simulink model "task1_sim"  (R2024a)
settings: Solver=VariableStepAuto  StartTime=0.0  StopTime=10.0  RelTol=1e-3
values from neighbouring files (symbols this model uses):
  a = zad1.a    [initilize_task1.m]    (also in task1.m; task1_1.m; task1_2.m; task1_3.m)
  b = zad1.b    [initilize_task1.m]    (also in task1.m; task1_1.m; task1_2.m; task1_3.m)
  Td = 0.1    [initilize_task1.m]    (also in task1.m; task1_1.m; task1_2.m; task1_3.m)
  w = zad1.w    [initilize_task1.m]    (also in task1.m; task1_1.m; task1_2.m; task1_3.m)
settings Model: Creator=ventus  LastModifiedBy=ventus

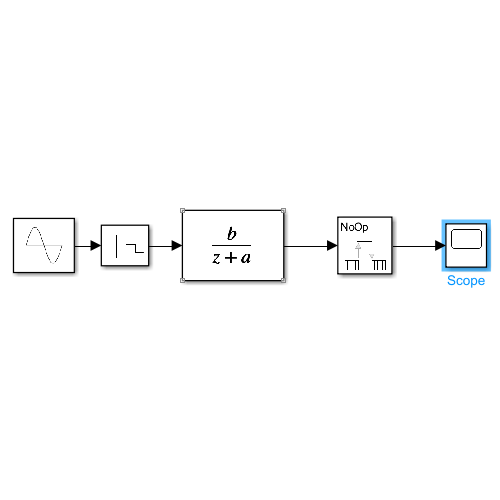
[thumbnail: Simulink's stored preview of the top-level diagram]
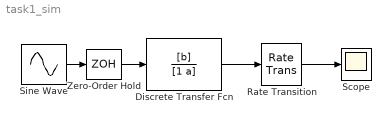
== system task1_sim ==
  Discrete Transfer Fcn : DiscreteTransferFcn  Numerator=[b]  Denominator=[1 a]
  Rate Transition : RateTransition  OutPortSampleTime=Td
  Scope : Scope
  Sine Wave : Sin  Frequency=w  SampleTime=0
  Zero-Order Hold : ZeroOrderHold  SampleTime=Td
  wires:
  Discrete Transfer Fcn/1 -> Rate Transition/1
  Rate Transition/1 -> Scope/1
  Sine Wave/1 -> Zero-Order Hold/1
  Zero-Order Hold/1 -> Discrete Transfer Fcn/1
